simulink model "Problem5"  (R2020b)
settings: Solver=VariableStepAuto  StartTime=0.0  StopTime=10  RelTol=1e-3
model workspace (MAT data in the model file):
  C = 25
  R = 20
settings Model: OrderedModelArguments=off  Creator=Administrator  LastModifiedBy=Administrator

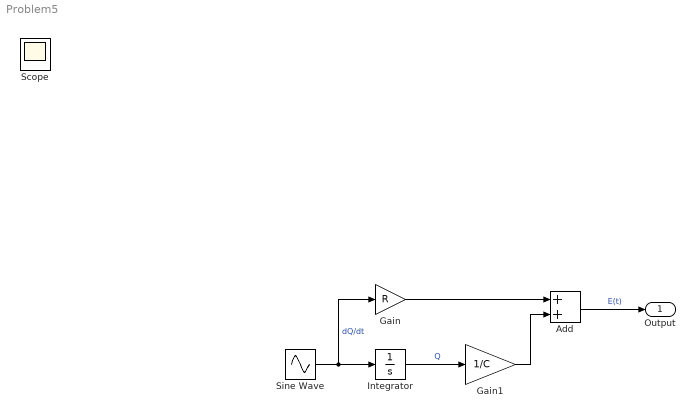
== system Problem5 ==
  Add : Sum
  Gain : Gain  Gain=R
  Gain1 : Gain  Gain=1/C
  Integrator : Integrator
  Sine Wave : Sin  SampleTime=0
  Output : Outport
  Scope : Scope
  wires:
  Integrator/1 -> Gain1/1  "Q"
  Gain1/1 -> Add/2
  Sine Wave/1 -> Integrator/1, Gain/1  "dQ/dt"
  Add/1 -> Output/1  "E(t)"
  Gain/1 -> Add/1
